simulink model "EulerSolver_Current_20161229"  (R2016a)
settings: Solver=ode45  StartTime=0.0  StopTime=20  MaxStep=0.001  RelTol=1e-5  AbsTol=1e-5
values from neighbouring files (symbols this model uses):
  I = [3 3 7]    [EulerSolverVariables_Current_20161229.m]
  N = [0 0 0]    [EulerSolverVariables_Current_20161229.m]
  w = [1 0 5]    [EulerSolverVariables_Current_20161229.m]
settings Model: Creator=Kevin  LastModifiedBy=Kevin
settings GRTTargetCC: GeneratePreprocessorConditionals=Use local settings
settings SimscapeCC: SimscapeLogType=all  SimscapeLogDataHistory=10000

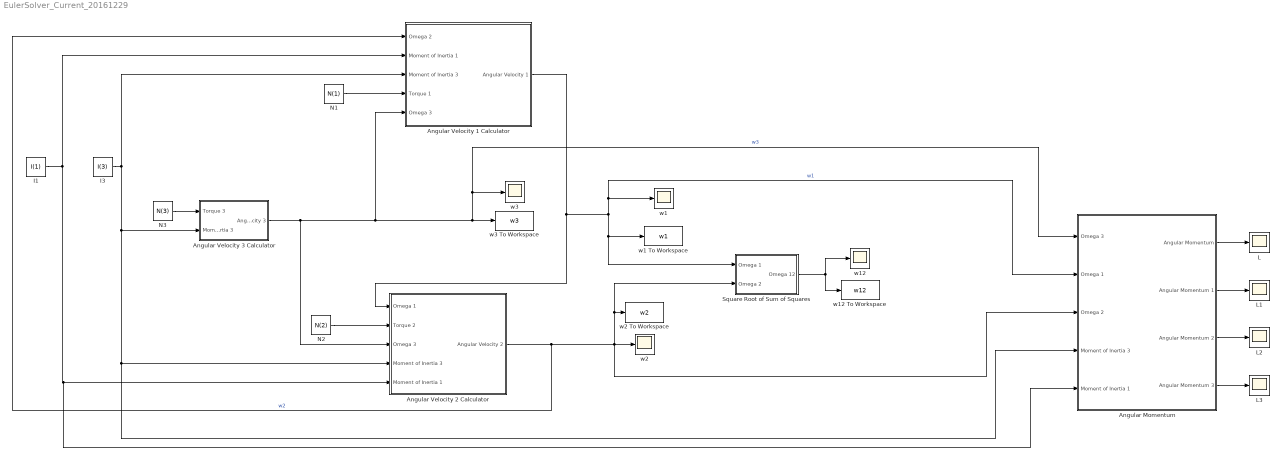
== system EulerSolver_Current_20161229 ==
  Angular Momentum : Subsystem
  Angular Velocity 1 Calculator : Subsystem
  Angular Velocity 2 Calculator : Subsystem
  Angular Velocity 3 Calculator : Subsystem
  I1 : Constant  Value=I(1)
  I3 : Constant  Value=I(3)
  L{,1..3} (4 alike) : Scope
  N1 : Constant  Value=N(1)
  N2 : Constant  Value=N(2)
  N3 : Constant  Value=N(3)
  Square Root of Sum of Squares : Subsystem
  w{1..3,12} (4 alike) : Scope
  w1 To Workspace : ToWorkspace  VariableName=w1  SaveFormat=Timeseries  SampleTime=-1
  w12 To Workspace : ToWorkspace  VariableName=w12  SaveFormat=Timeseries  SampleTime=-1
  w2 To Workspace : ToWorkspace  VariableName=w2  SaveFormat=Timeseries  SampleTime=-1
  w3 To Workspace : ToWorkspace  VariableName=w3  SaveFormat=Timeseries  SampleTime=-1
  wires:
  Angular Velocity 3 Calculator/1("Angular Velocity 3 ") -> Angular Velocity 1 Calculator/5(Omega 3), Angular Momentum/1(Omega 3), w3/1, w3 To Workspace/1, Angular Velocity 2 Calculator/3(Omega 3)  "w3"
  Angular Momentum/1(Angular Momentum) -> L/1
  Angular Momentum/2(Angular Momentum 1) -> L1/1
  Angular Momentum/3(Angular Momentum 2) -> L2/1
  Angular Momentum/4(Angular Momentum 3) -> L3/1
  N3/1 -> Angular Velocity 3 Calculator/1(Torque 3)
  I3/1 -> Angular Velocity 1 Calculator/3(Moment of Inertia 3), Angular Momentum/4(Moment of Inertia 3), Angular Velocity 2 Calculator/4(Moment of Inertia 3), Angular Velocity 3 Calculator/2(Moment of Inertia 3)
  Angular Velocity 1 Calculator/1(Angular Velocity 1) -> Square Root of Sum of Squares/1(Omega 1), w1 To Workspace/1, Angular Momentum/2(Omega 1), w1/1, Angular Velocity 2 Calculator/1(Omega 1)  "w1"
  N1/1 -> Angular Velocity 1 Calculator/4(Torque 1)
  I1/1 -> Angular Velocity 1 Calculator/2(Moment of Inertia 1), Angular Momentum/5("Moment of Inertia 1 "), Angular Velocity 2 Calculator/5(Moment of Inertia 1)
  Angular Velocity 2 Calculator/1(Angular Velocity 2) -> Angular Momentum/3(Omega 2), w2/1, Square Root of Sum of Squares/2(Omega 2), w2 To Workspace/1, Angular Velocity 1 Calculator/1(Omega 2)  "w2"
  N2/1 -> Angular Velocity 2 Calculator/2(Torque 2)
  Square Root of Sum of Squares/1(Omega 12) -> w12 To Workspace/1, w12/1

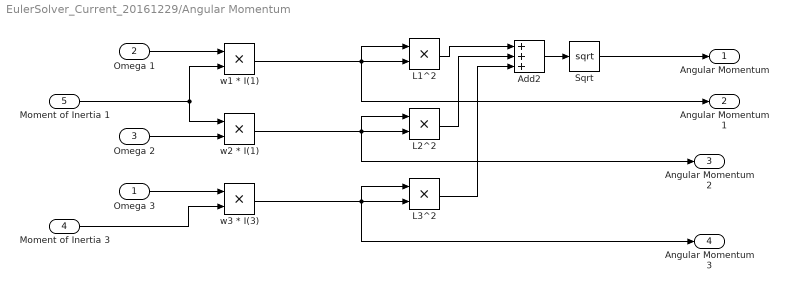
== system EulerSolver_Current_20161229/Angular Momentum ==
  Omega 3 : Inport
  Omega 1 : Inport  Port=2
  Omega 2 : Inport  Port=3
  Moment of Inertia 3 : Inport  Port=4
  "Moment of Inertia 1 " : Inport  Port=5
  Add2 : Sum  Inputs=+++
  L1^2 : Product
  L2^2 : Product
  L3^2 : Product
  Sqrt : Sqrt  SaturateOnIntegerOverflow=on
  w1 * I(1) : Product
  w2 * I(1) : Product
  w3 * I(3) : Product
  Angular Momentum : Outport
  Angular Momentum 1 : Outport  Port=2
  Angular Momentum 2 : Outport  Port=3
  Angular Momentum 3 : Outport  Port=4
  wires:
  w2 * I(1)/1 -> Angular Momentum 2/1, L2^2/2, L2^2/1
  L1^2/1 -> Add2/1
  Sqrt/1 -> Angular Momentum/1
  L3^2/1 -> Add2/3
  Add2/1 -> Sqrt/1
  L2^2/1 -> Add2/2
  w3 * I(3)/1 -> Angular Momentum 3/1, L3^2/2, L3^2/1
  w1 * I(1)/1 -> Angular Momentum 1/1, L1^2/1, L1^2/2
  Omega 3/1 -> w3 * I(3)/1
  Omega 2/1 -> w2 * I(1)/2
  Omega 1/1 -> w1 * I(1)/1
  Moment of Inertia 3/1 -> w3 * I(3)/2
  "Moment of Inertia 1 "/1 -> w1 * I(1)/2, w2 * I(1)/1

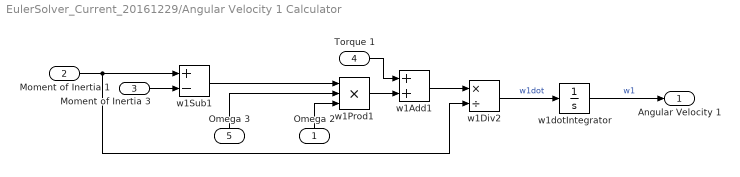
== system EulerSolver_Current_20161229/Angular Velocity 1 Calculator ==
  Omega 2 : Inport
  Moment of Inertia 1 : Inport  Port=2
  Moment of Inertia 3 : Inport  Port=3
  Torque 1 : Inport  Port=4
  Omega 3 : Inport  Port=5
  w1Add1 : Sum
  w1Div2 : Product  Inputs=*/
  w1Prod1 : Product  Inputs=3
  w1Sub1 : Sum  Inputs=+-
  w1dotIntegrator : Integrator  InitialCondition=w(1)
  Angular Velocity 1 : Outport
  wires:
  Torque 1/1 -> w1Add1/1
  w1Prod1/1 -> w1Add1/2
  w1dotIntegrator/1 -> Angular Velocity 1/1  "w1"
  w1Div2/1 -> w1dotIntegrator/1  "w1dot"
  w1Sub1/1 -> w1Prod1/1
  Omega 3/1 -> w1Prod1/2
  Omega 2/1 -> w1Prod1/3
  Moment of Inertia 3/1 -> w1Sub1/2
  Moment of Inertia 1/1 -> w1Div2/2, w1Sub1/1
  w1Add1/1 -> w1Div2/1

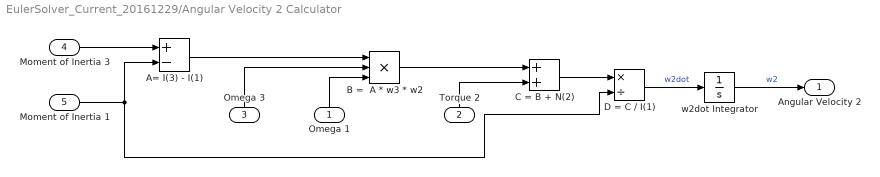
== system EulerSolver_Current_20161229/Angular Velocity 2 Calculator ==
  Omega 1 : Inport
  Torque 2 : Inport  Port=2
  Omega 3 : Inport  Port=3
  Moment of Inertia 3 : Inport  Port=4
  Moment of Inertia 1 : Inport  Port=5
  A= I(3) - I(1) : Sum  Inputs=+-
  B =  A * w3 * w2 : Product  Inputs=3
  C = B + N(2) : Sum
  D = C / I(1) : Product  Inputs=*/
  w2dot Integrator : Integrator  InitialCondition=w(2)
  Angular Velocity 2 : Outport
  wires:
  D = C / I(1)/1 -> w2dot Integrator/1  "w2dot"
  Torque 2/1 -> C = B + N(2)/2
  B =  A * w3 * w2/1 -> C = B + N(2)/1
  C = B + N(2)/1 -> D = C / I(1)/1
  w2dot Integrator/1 -> Angular Velocity 2/1  "w2"
  A= I(3) - I(1)/1 -> B =  A * w3 * w2/1
  Omega 1/1 -> B =  A * w3 * w2/3
  Moment of Inertia 3/1 -> A= I(3) - I(1)/1
  Moment of Inertia 1/1 -> A= I(3) - I(1)/2, D = C / I(1)/2
  Omega 3/1 -> B =  A * w3 * w2/2

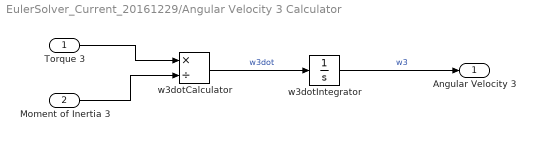
== system EulerSolver_Current_20161229/Angular Velocity 3 Calculator ==
  Torque 3 : Inport
  Moment of Inertia 3 : Inport  Port=2
  w3dotCalculator : Product  Inputs=*/
  w3dotIntegrator : Integrator  InitialCondition=w(3)
  "Angular Velocity 3 " : Outport
  wires:
  w3dotIntegrator/1 -> "Angular Velocity 3 "/1  "w3"
  w3dotCalculator/1 -> w3dotIntegrator/1  "w3dot"
  Torque 3/1 -> w3dotCalculator/1
  Moment of Inertia 3/1 -> w3dotCalculator/2

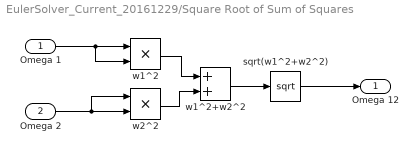
== system EulerSolver_Current_20161229/Square Root of Sum of Squares ==
  Omega 1 : Inport
  Omega 2 : Inport  Port=2
  sqrt(w1^2+w2^2) : Sqrt  SaturateOnIntegerOverflow=on
  w1^2 : Product
  w1^2+w2^2 : Sum
  w2^2 : Product
  Omega 12 : Outport
  wires:
  w1^2+w2^2/1 -> sqrt(w1^2+w2^2)/1
  sqrt(w1^2+w2^2)/1 -> Omega 12/1
  w2^2/1 -> w1^2+w2^2/2
  w1^2/1 -> w1^2+w2^2/1
  Omega 1/1 -> w1^2/2, w1^2/1
  Omega 2/1 -> w2^2/1, w2^2/2
